simulink model "vidu04"  (R2016a)
settings: Solver=VariableStepAuto  StartTime=0.0  StopTime=8000  RelTol=1e-3
settings Model: Creator=Lenovo  LastModifiedBy=Lenovo

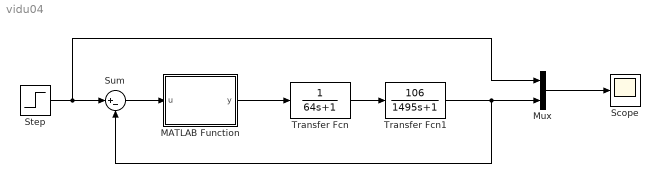
== system vidu04 ==
  MATLAB Function : MATLAB Function  TreatAsAtomicUnit=on
  Mux : Mux  Inputs=2
  Scope : Scope
  Step : Step  Time=0  After=100  SampleTime=0
  Sum : Sum  Inputs=|+-
  Transfer Fcn : TransferFcn  Denominator=[64 1]
  Transfer Fcn1 : TransferFcn  Numerator=[106]  Denominator=[1495 1]
  wires:
  Mux/1 -> Scope/1
  Step/1 -> Mux/1, Sum/1
  Sum/1 -> MATLAB Function/1(u)
  Transfer Fcn/1 -> Transfer Fcn1/1
  Transfer Fcn1/1 -> Mux/2, Sum/2
  MATLAB Function/1(y) -> Transfer Fcn/1

== matlab function vidu04/MATLAB Function ==
  data: u input; y output
function y = relay(u)
%#codegen
   D = 1;
   sw = 1;
   
   if abs(u) >= D
       y = sw*sign(u);
   else
       y = -sw*sign(diff(u));
   end
   
end
